simulink model "GeneralFramework"  (R2022a)
settings: Solver=ode23tb  StartTime=0.0  StopTime=t_sim  RelTol=1e-3
values from neighbouring files (symbols this model uses):
  AccPwrbp = [0 3.0779560993538198]    [Init_Parameters.m]
  AccSpdbp = [256.49641719585139 641.24104298962845]    [Init_Parameters.m]
  EngTrqSat = 60    [Init_Parameters.m]
  f_mu = ones(4,1)    [Init_Parameters.m]
  InitialLatPosition = 0    [Init_Parameters.m]
  numWheels = 4    [Init_Parameters.m]    (also in VehicleParameters.m)
  omega_hw = 13.51    [Init_Parameters.m]
  steerDir = -1    [Init_Parameters.m]
  t_start = 1    [Init_Parameters.m]
  t_stop = 100    [Init_Parameters.m]
  theta_max = 270    [Init_Parameters.m]
  TrackWidth = VEH.TrackWidth    [Init_Parameters.m]
  Trans = data.Trans    [Init_Parameters.m]    (also in ModelWorkspace.mat = )
  VEH = data.VEH    [Init_Parameters.m]    (also in ModelWorkspace.mat = ; VehicleParameters.m)
  wheelB = VEH.FrontAxlePositionfromCG+VEH.RearAxlePositionfromCG    [Init_Parameters.m]    (also in VehicleParameters.m)
  xdot_r = 2    [Init_Parameters.m]
libraries: autolibutils x10, simulink x8, sharedtransform x5, autolibsharedcoupling x3, vehdynlibsuspension x2, shared6dof x2, autolibtranscontrolscommon x1, vehdynlibdriver x1, autolibsharedtransfixedgear x1, vehdynlibsteering x1, autolibshareddiff x1, autolibsharedmappedengines x1
(part 1 of 5)
settings Model: Creator=monic  LastModifiedBy=monic
settings DebuggingCC: UnconnectedInputMsg=warning  UnconnectedOutputMsg=warning  UnconnectedLineMsg=warning
settings RTWCC: DLArmComputeVersion=19.05

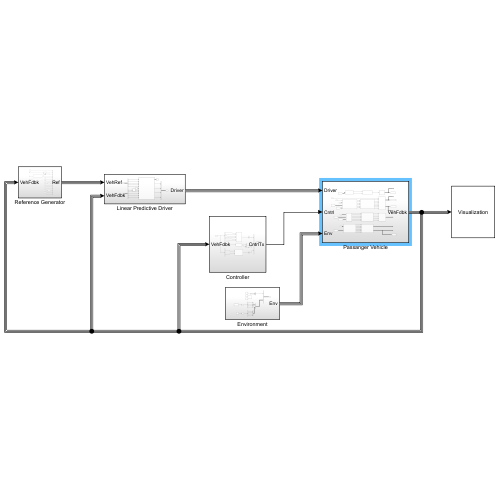
[thumbnail: Simulink's stored preview of the top-level diagram]
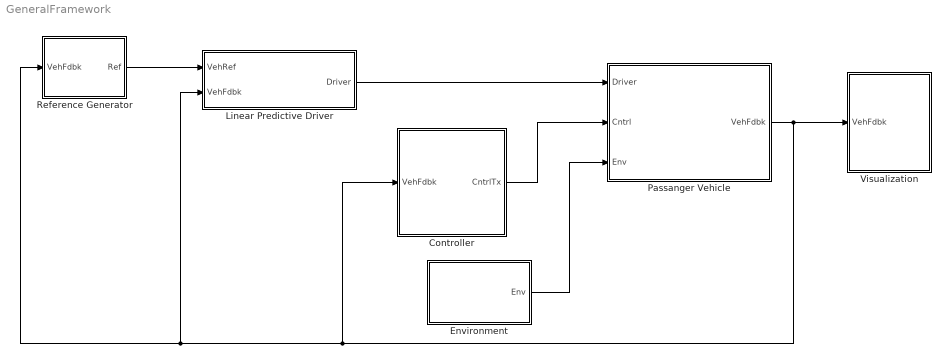
== system GeneralFramework ==
  Controller : Subsystem
  Environment : Subsystem
  Linear Predictive Driver : Subsystem
  Passanger Vehicle : Subsystem
  Reference Generator : Subsystem
  Visualization : Subsystem
      mask Display: disp('Visualization')
  wires:
  Environment/1(Env) -> Passanger Vehicle/3(Env)
  Linear Predictive Driver/1(Driver) -> Passanger Vehicle/1(Driver)
  Passanger Vehicle/1(VehFdbk) -> Visualization/1(VehFdbk), Controller/1(VehFdbk), Linear Predictive Driver/2(VehFdbk), Reference Generator/1(VehFdbk)
  Reference Generator/1(Ref) -> Linear Predictive Driver/1(VehRef)
  Controller/1(CntrlTx) -> Passanger Vehicle/2(Cntrl)

== system GeneralFramework/Controller ==
  VehFdbk : Inport
  Active Differential Control : Subsystem  VariantControl=0
  Brake Pressure Control : Subsystem  VariantControl=0
  Bus Creator1 : BusCreator  Inputs=1
  Bus Creator2 : BusCreator  Inputs=2
  Bus Creator3 : BusCreator  Inputs=3
  Bus Creator4 : BusCreator  Inputs=1
  Bus Selector : BusSelector  OutputSignals=Driver.DecelFdbk
  Bus Selector1 : BusSelector  OutputSignals=Driver.AccFdbk,Driver.DecelFdbk,Driver.GearFdbk,Driveline.EngSpd,Wheels.TireFrame.Omega
  Bus Selector3 : BusSelector  OutputSignals=Driver.AccFdbk,Driver.SteerFdbk
  Trasmission Control : Subsystem
  CntrlTx : Outport  VectorParamsAs1DForOutWhenUnconnected=off
  wires:
  VehFdbk/1 -> Bus Selector3/1, Bus Selector/1, Bus Selector1/1
  Bus Selector1/3 -> Trasmission Control/3(GearReq)  "<GearFdbk>"
  Bus Selector1/4 -> Trasmission Control/4(EngSpd)  "<EngSpd>"
  Bus Selector1/2 -> Trasmission Control/2(BrkCmd)  "<DecelFdbk>"
  Bus Selector1/5 -> Trasmission Control/5(Omega)  "<Omega>"
  Bus Selector/1 -> ?  "<DecelFdbk>"
  Bus Selector1/1 -> Trasmission Control/1(Accel)  "<AccFdbk>"
  [ABSFlag] -> Trasmission Control/6(ABSFlag)
  Bus Selector3/2 -> Active Differential Control/2(Steer)  "<SteerFdbk>"
  Bus Selector3/1 -> Active Differential Control/1(axayaz)  "<AccFdbk>"
  Brake Pressure Control/2(ABSFlag) -> [ABSFlag], Bus Creator2/2  "ABSFlag"
  Brake Pressure Control/1(BrkPrsCmd) -> Bus Creator2/1  "BrkPrsCmd"
  Bus Creator3/1 -> CntrlTx/1  "CntrlTx"
  Trasmission Control/1(Gear) -> Bus Creator1/1  "GearCmd"
  Active Differential Control/1(DiffPrsCmd) -> Bus Creator4/1  "DiffPrsCmd"
  Bus Creator4/1 -> Bus Creator3/3  "Diff"
  Bus Creator1/1 -> Bus Creator3/1  "Transmission"
  Bus Creator2/1 -> Bus Creator3/2  "BrkPrsCmd"

== system GeneralFramework/Environment ==
  Bus Creator : BusCreator  Inputs=4
  Bus Creator1 : BusCreator  Inputs=2
  Bus Creator2 : BusCreator  Inputs=4
  Bus Creator3 : BusCreator  Inputs=2
  Constant1 : Constant  Value=zeros(4,1)
  Constant2 : Constant  Value=f_mu
  Constant3 : Constant  Value=0
  Constant4 : Constant  Value=0
  Constant5 : Constant  Value=0
  Demux : Demux
  Demux1 : Demux
  Signal Specification : SignalSpecification  Unit=m
  Signal Specification1 : SignalSpecification  Unit=1
  Vector Concatenate : Concatenate  NumInputs=3
  Env : Outport  VectorParamsAs1DForOutWhenUnconnected=off
  wires:
  Constant3/1 -> Vector Concatenate/1  "X"
  Constant5/1 -> Vector Concatenate/3  "Z"
  Bus Creator1/1 -> Env/1
  Vector Concatenate/1 -> Bus Creator1/1  "Wind"
  Constant4/1 -> Vector Concatenate/2  "Y"
  Bus Creator3/1 -> Bus Creator1/2  "Ground"
  Demux1/3 -> Bus Creator2/3  "mu_RL"
  Demux1/1 -> Bus Creator2/1  "mu_FL"
  Bus Creator2/1 -> Bus Creator3/2  "mu"
  Demux1/4 -> Bus Creator2/4  "mu_RR"
  Bus Creator/1 -> Bus Creator3/1  "z"
  Demux1/2 -> Bus Creator2/2  "mu_FR"
  Demux/2 -> Bus Creator/2  "G_FR_z"
  Signal Specification1/1 -> Demux1/1
  Demux/3 -> Bus Creator/3  "G_RL_z"
  Demux/4 -> Bus Creator/4  "G_RR_z"
  Demux/1 -> Bus Creator/1  "G_FL_z"
  Signal Specification/1 -> Demux/1
  Constant1/1 -> Signal Specification/1
  Constant2/1 -> Signal Specification1/1

== system GeneralFramework/Linear Predictive Driver ==
  VehRef : Inport
  VehFdbk : Inport  Port=2
  Bus Creator1 : BusCreator  Inputs=4
  Bus Selector : BusSelector  OutputSignals=Body.BdyFrm.Cg.Vel.xdot,Body.InertFrm.Cg.Disp.Y,Body.BdyFrm.Cg.Vel.ydot,Body.InertFrm.Cg.Ang.psi,Body.BdyFrm.Cg.AngVel.r
  Bus Selector1 : BusSelector  OutputSignals=LngRef,LtrlRef,EnblSteerCmd,SteerOvrCmd,AccelZero
  Dead Zone : DeadZone  LowerValue=-.5  UpperValue=.5  ZeroCross=off
  Ground : Ground
  Linear Predictive Driver : vehdynlibdriver/Predictive Driver  extAccelOvr=off  extDecelOvr=off  extAccelHld=off  extDecelHld=off  extAccelZero=on  extDecelZero=off  extSteerOvr=on  extSteerHld=off  extSteerZero=off  cntrlType=Predictive  cntrlTypeLat=Predictive  shftType=Reverse, Neutral, Drive  coordMode=SAE J670 (Z-down)  refType=Reference pose  velUnits=m/s  angUnits=rad  gearOut=on  steerOut=on  Kp=3  Ki=1  Kff=1  Kg=0  VehVelVec=[0 100]  KffVec=[.1 .1]  KpVec=[10 10]  KiVec=[5 5]  KgVec=[0 0]  vnom=5  Kaw=1  tauerr=.075  tau=0.3  L=0.75  Kpt=15000  aR=200  bR=2.5  cR=.5  g=9.81  vecPose=off  dynamMode=off  PositionGainF=2.5  PositionGainR=2.5  YawRateGain=.2  DelayGain=.2  enableDrift=off  BetaRef=20*pi/180  KpBeta=1  KpDrift=2  KdDrift=1  KpPsi=6  KOmega=30  tOmega=1  a=VEH.FrontAxlePositionfromCG  b=VEH.RearAxlePositionfromCG  m=VEH.Mass  Cy_f=50000  Cy_r=70000  I=VEH.YawMomentInertia  Ksteer=18  theta=40*pi/180  Idl=3  Re=.3  lambda_mu=1  GearInit=0  tShift=.1  pdlVec=[0.1 0.4 0.5 0.9]  upShftTbl=[-1 12.9375 26.4375 39.9375 51.18749999999999 62.4375 72.84375 83.25;-1 16.3125 29.8125 43.3125 54.5624 65.8125 76.78125 87.75;-1 19.6875 33.1875 46.68749999999999 57.9375 69.1875 80.71875 92.25;-1 33 52.5 77.25 100.5 138.75 161.875 185]  dwnShftTbl=[-1 12.9375 26.4375 39.9375 51.18749999999999 62.4375 72.84375 83.25;-1 16.3125 29.8125 43.3125 54.5624 65.8125 76.78125 87.75;-1 19.6875 33.1875 46.68749999999999 57.9375 69.1875 80.71875 92.25;-1 33 52.5 77.25 100.5 138.75 161.875 185]  tClutch=.5  tRev=.5  tPark=120  UpGearVec="[0  1  2  3  4  5  6  7]"  DownGearVec="[1  2  3  4  5  6  7  8]"  aMode=2
      settings: SourceProductBaseCode=VE
  Terminator : Terminator
  Driver : Outport
  wires:
  Linear Predictive Driver/4 -> Bus Creator1/3  "DecelCmd"
  Bus Selector/3 -> Linear Predictive Driver/9  "<ydot>"
  Ground/1 -> Linear Predictive Driver/6
  Bus Selector/5 -> Linear Predictive Driver/11  "<r>"
  VehFdbk/1 -> Bus Selector/1
  Bus Selector1/4 -> Linear Predictive Driver/4  "<SteerOvrCmd>"
  Bus Selector/1 -> Dead Zone/1  "<xdot>"
  Bus Selector1/1 -> Linear Predictive Driver/1  "<LngRef>"
  Bus Selector1/2 -> Linear Predictive Driver/2  "<LtrlRef>"
  Linear Predictive Driver/3 -> Bus Creator1/2  "AccelCmd"
  Bus Selector1/3 -> Linear Predictive Driver/3  "<EnblSteerCmd>"
  Linear Predictive Driver/5 -> Bus Creator1/4  "GearCmd"
  Bus Creator1/1 -> Driver/1
  Bus Selector/2 -> Linear Predictive Driver/8  "<Y>"
  Linear Predictive Driver/2 -> Bus Creator1/1  "SteerCmd"
  Bus Selector/4 -> Linear Predictive Driver/10  "<psi>"
  Bus Selector1/5 -> Linear Predictive Driver/5  "<AccelZero>"
  Linear Predictive Driver/1 -> Terminator/1
  Dead Zone/1 -> Linear Predictive Driver/7
  VehRef/1 -> Bus Selector1/1

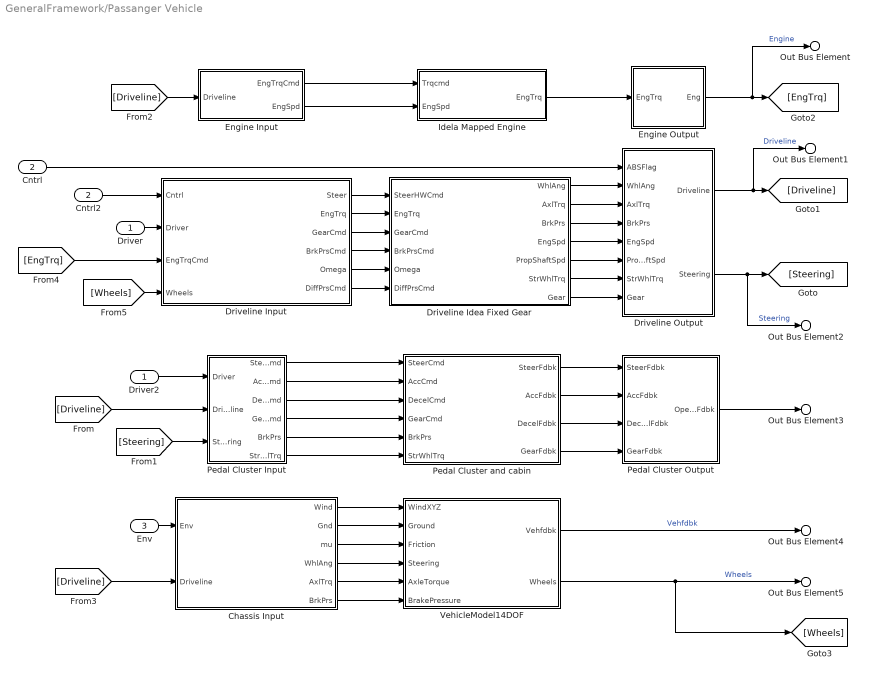
== system GeneralFramework/Passanger Vehicle ==
  Driver : Inport
  Cntrl : Inport  Port=2
  Env : Inport  Port=3
  Chassis Input : Subsystem
  Cntrl2 : InportShadow  Port=2
  Driveline Idea Fixed Gear : Subsystem
  Driveline Input : Subsystem
  Driveline Output : Subsystem
  Driver2 : InportShadow
  Engine Input : Subsystem
  Engine Output : Subsystem
  Idela Mapped Engine : Subsystem
  Pedal Cluster Input : Subsystem
  Pedal Cluster Output : Subsystem
  Pedal Cluster and cabin : Subsystem
  VehicleModel14DOF : Subsystem
  Out Bus Element4 : Outport  PortName=VehFdbk  Element=Body
  Out Bus Element5 : Outport  PortName=VehFdbk  Element=Wheels
  Out Bus Element3 : Outport  PortName=VehFdbk  Element=Driver
  Out Bus Element2 : Outport  PortName=VehFdbk  Element=Steering
  Out Bus Element1 : Outport  PortName=VehFdbk  Element=Driveline
  Out Bus Element : Outport  PortName=VehFdbk  Element=Engine
  wires:
  Driveline Idea Fixed Gear/7(Gear) -> Driveline Output/8(Gear)
  [Driveline] -> Chassis Input/2(Driveline)
  Engine Input/1(EngTrqCmd) -> Idela Mapped Engine/1(Trqcmd)
  Pedal Cluster and cabin/2(AccFdbk) -> Pedal Cluster Output/2(AccFdbk)
  Driveline Input/4(BrkPrsCmd) -> Driveline Idea Fixed Gear/4(BrkPrsCmd)
  Pedal Cluster Input/3(DecelCmd) -> Pedal Cluster and cabin/3(DecelCmd)
  VehicleModel14DOF/2(Wheels) -> Out Bus Element5/1, [Wheels]  "Wheels"
  Pedal Cluster Input/2(AccelCmd) -> Pedal Cluster and cabin/2(AccCmd)
  Driver/1 -> Driveline Input/2(Driver)
  Pedal Cluster and cabin/3(DecelFdbk) -> Pedal Cluster Output/3(DecelFdbk)
  Engine Input/2(EngSpd) -> Idela Mapped Engine/2(EngSpd)
  [Driveline] -> Pedal Cluster Input/2(Driveline)
  Driveline Idea Fixed Gear/1(WhlAng) -> Driveline Output/2(WhlAng)
  Pedal Cluster and cabin/4(GearFdbk) -> Pedal Cluster Output/4(GearFdbk)
  Driveline Input/3(GearCmd) -> Driveline Idea Fixed Gear/3(GearCmd)
  [Steering] -> Pedal Cluster Input/3(Steering)
  Cntrl/1 -> Driveline Output/1(ABSFlag)
  [EngTrq] -> Driveline Input/3(EngTrqCmd)
  Driveline Input/6(DiffPrsCmd) -> Driveline Idea Fixed Gear/6(DiffPrsCmd)
  Driver2/1 -> Pedal Cluster Input/1(Driver)
  Idela Mapped Engine/1(EngTrq) -> Engine Output/1("EngTrq ")
  Pedal Cluster Input/1(SteerCmd) -> Pedal Cluster and cabin/1(SteerCmd)
  Pedal Cluster Input/5(BrkPrs) -> Pedal Cluster and cabin/5(BrkPrs)
  [Wheels] -> Driveline Input/4(Wheels)
  Driveline Input/1(Steer) -> Driveline Idea Fixed Gear/1(SteerHWCmd)
  Driveline Input/2(EngTrq) -> Driveline Idea Fixed Gear/2(EngTrq)
  Pedal Cluster and cabin/1(SteerFdbk) -> Pedal Cluster Output/1(SteerFdbk)
  Driveline Input/5(Omega) -> Driveline Idea Fixed Gear/5(Omega)
  Env/1 -> Chassis Input/1(Env)
  Driveline Idea Fixed Gear/3(BrkPrs) -> Driveline Output/4(BrkPrs)
  Driveline Idea Fixed Gear/4(EngSpd) -> Driveline Output/5(EngSpd)
  Driveline Output/2(Steering) -> Out Bus Element2/1, [Steering]  "Steering"
  Engine Output/1(Eng) -> Out Bus Element/1, [EngTrq]  "Engine"
  Driveline Idea Fixed Gear/6(StrWhlTrq) -> Driveline Output/7(StrWhlTrq)
  Driveline Idea Fixed Gear/5(PropShaftSpd) -> Driveline Output/6(PropShftSpd)
  [Driveline] -> Engine Input/1(Driveline)
  Pedal Cluster Input/4(GearCmd) -> Pedal Cluster and cabin/4(GearCmd)
  Driveline Idea Fixed Gear/2(AxlTrq) -> Driveline Output/3(AxlTrq)
  VehicleModel14DOF/1(Vehfdbk) -> Out Bus Element4/1  "Vehfdbk"
  Pedal Cluster Input/6(StrWhlTrq) -> Pedal Cluster and cabin/6(StrWhlTrq)
  Cntrl2/1 -> Driveline Input/1(Cntrl)
  Pedal Cluster Output/1(OperatorFdbk) -> Out Bus Element3/1
  Driveline Output/1(Driveline) -> Out Bus Element1/1, [Driveline]  "Driveline"
  Chassis Input/1(Wind) -> VehicleModel14DOF/1(WindXYZ)
  Chassis Input/2(Gnd) -> VehicleModel14DOF/2(Ground)
  Chassis Input/3(mu) -> VehicleModel14DOF/3(Friction)
  Chassis Input/4(WhlAng) -> VehicleModel14DOF/4(Steering)
  Chassis Input/5(AxlTrq) -> VehicleModel14DOF/5(AxleTorque)
  Chassis Input/6(BrkPrs) -> VehicleModel14DOF/6(BrakePressure)

== system GeneralFramework/Reference Generator ==
  Bus Element In1 : Inport  PortName=VehFdbk  Element=Body.BdyFrm.Cg.Vel.xdot
  Bus Element In2 : Inport  PortName=VehFdbk  Element=Body.InertFrm.Cg.Disp.Y
  Bus Creator2 : BusCreator  Inputs=14
  Compare To Zero : simulink/Logic and Bit Operations/Compare To Zero  relop=~=  OutDataTypeStr=boolean  ZeroCross=off
  Constant{4..7,10..12} (7 alike) : Constant  Value=false
  Constant2 : Constant  Value=false  OutDataTypeStr=boolean
  Constant3 : Constant  Value=0
  Constant8 : Constant  Value=0
  Ground : Ground
  LatchSwitchCont : autolibutils/LatchSwitchCont  aMode=2
      settings: SourceProductBaseCode=PW,DR,MT,VE
  Longitudinal Velocity Reference : vehdynlibscenariocommon/Slowly Increasing Steer/Longitudinal Velocity Reference  SystemSampleTime=-1  VariantActivationTime=update diagram  Latency=0  AutoFrameSizeCalculation=off
      settings: SourceProductBaseCode=VE
  Signal Specification : SignalSpecification  Unit=m
  Signal Specification2 : SignalSpecification  Unit=one
  Signal Specification3 : SignalSpecification  Unit=one
  Steer Command Generator : Subsystem
  Ref : Outport  VectorParamsAs1DForOutWhenUnconnected=off
  wires:
  Steer Command Generator/1(SteerOvrCmd) -> Compare To Zero/1, Bus Creator2/4  "SteerOvrCmd"
  Signal Specification3/1 -> Bus Creator2/12  "DecelOvrCmd"
  Constant10/1 -> Bus Creator2/11  "EnblDecelCmd"
  Constant4/1 -> Bus Creator2/7  "EnblAccelOvr"
  LatchSwitchCont/1 -> Bus Creator2/3  "EnblSteerCmd"
  Constant8/1 -> Signal Specification2/1
  Signal Specification2/1 -> Bus Creator2/8  "AccelOvrCmd"
  Longitudinal Velocity Reference/1 -> Bus Creator2/1  "LngRef"
  Constant3/1 -> Signal Specification3/1
  Bus Creator2/1 -> Ref/1
  Constant2/1 -> Bus Creator2/10  "AccelZero"
  Constant5/1 -> Bus Creator2/5  "SteerHld"
  Compare To Zero/1 -> LatchSwitchCont/1
  Constant7/1 -> Bus Creator2/9  "AccelHld"
  Signal Specification/1 -> Bus Creator2/2  "LtrlRef"
  Constant6/1 -> Bus Creator2/6  "SteerZero"
  Constant11/1 -> Bus Creator2/13  "DecelHld"
  Constant12/1 -> Bus Creator2/14  "DecelZero"
  Ground/1 -> LatchSwitchCont/2
  Bus Element In1/1 -> Steer Command Generator/1(<xdot>)
  Bus Element In2/1 -> Signal Specification/1

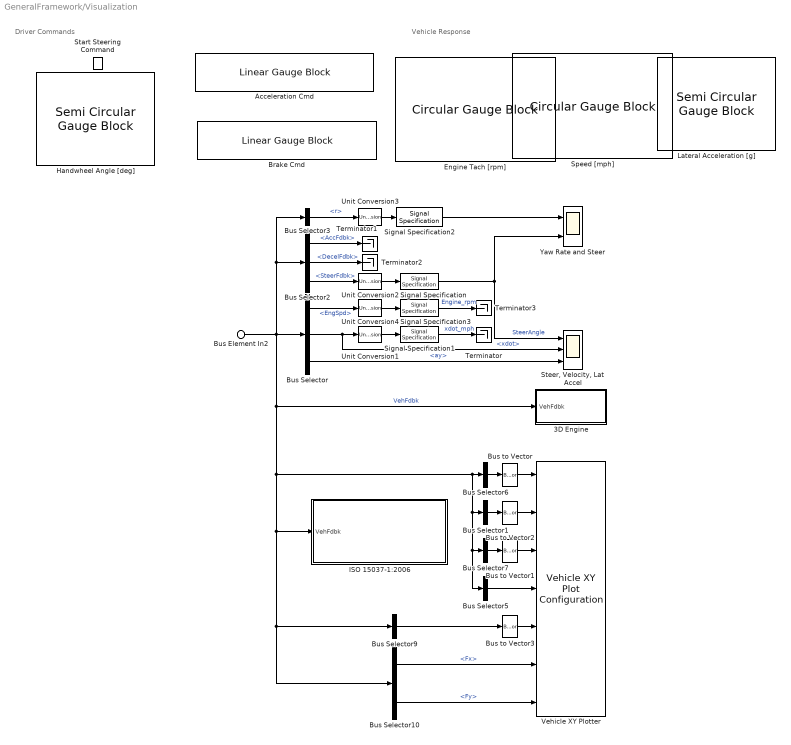
== system GeneralFramework/Visualization ==
  note: Driver Commands
  note: Vehicle Response
  Bus Element In2 : Inport  PortName=VehFdbk
  3D Engine : Subsystem  Variant=on  mask(3D Engine){engine3D=Disabled, use3DOp=off, SceneDesc=Open surface, dt3D=.03, defaultPos=Recommended for scene, X_o=0, Y_o=0, Z_o=0, phi_o=0, theta_o=0, psi_o=0}
      mask prompts: engine3D "vdynblks:vehdynRefApp3DEng:blkPrm_engine3D"; use3DOp "Use default operating point"; SceneDesc "vdynblks:vehdynRefApp3DEng:blkPrm_SceneDesc"; dt3D "vdynblks:vehdynRefApp3DEng:blkPrm_dt3D"; X_o "vdynblks:vehdynRefApp3DEng:blkPrm_X_o"; Y_o "vdynblks:vehdynRefApp3DEng:blkPrm_Y_o"; Z_o "vdynblks:vehdynRefApp3DEng:blkPrm_Z_o"; phi_o "vdynblks:vehdynRefApp3DEng:blkPrm_phi_o"; theta_o "vdynblks:vehdynRefApp3DEng:blkPrm_theta_o"; psi_o "vdynblks:vehdynRefApp3DEng:blkPrm_psi_o"
      mask help: This subsystem contains the interface blocks which permit the display of the vehicle in the 3D virtual environment. Enable it to view the simulation progress, disable it to inhibit the display.
      mask init:
      | GrndFdbkPath = find_system(bdroot(gcb),'BlockType','SubSystem','Name','Ground Feedback');
      | ManBlkName = 'Slowly Increasing Steer';
      | ManBlkPath = find_system(bdroot(gcb),'BlockType','SubSystem','Name',ManBlkName);
      | OpVarName = 'dlcSS35mph';
      | switch get_param(gcb,'engine3D')    
      |     case 'Disabled'
      |         try
      |             set_param(GrndFdbkPath{:},'OverrideUsingVariant','0');
      |         catch
      |             disp('Warning: No ground feedback sensor not set')
      |         end
      |         try
      |             if strcmp(get_param(gcb,'use3DOp'),'on') && strcmp(get_param(ManBlkPath{:},'ssMode'),'Resume from a workspace variable')
      |                 set_param(ManBlkPath{:},'ssVar',OpVarName);
      |             end
      |         catch
      |              disp('Warning: Maneuver source block not found. Steady state operating point not set')
      |         end
      |     case 'Enabled'
      |         try
      |             set_param(GrndFdbkPath{:},'OverrideUsingVariant','1');            
      |         catch
      |             disp('Warning: Ground feedback from game engine was not found. Using constant values from model instead.')
      |         end
      |         try
      |             if strcmp(get_param(gcb,'use3DOp'),'on') && strcmp(get_param(ManBlkPath{:},'ssMode'),'Resume from a workspace variable')
      |                 set_param(ManBlkPath{:},'ssVar',[OpVarName '3D']);
      |             end
      |         catch
      |              disp('Warning: Maneuver source block not found. Steady state operating point not set')
      |         end
      |     otherwise
      | end
      settings: AttributesFormatString=|
      | %<SceneDesc>
      | %<engine3D>
      mask Help: eval('vdynblkshelp(''vdynblks3dengine'')');
      mask TypeOptions engine3D: Enabled | Disabled
      mask Callback engine3D:
      | switch get_param(gcb,'engine3D')
      |     case 'Disabled'
      |         try
      |             % add specifics here if needed
      |         catch
      |             disp('Warning: Maneuver source block not found in model')
      |         end
      |     case 'Enabled'
      |         try
      |             % add specifics here if needed
      |         catch
      |             disp('Warning: Maneuver source block not found in model')
      |         end
      |     otherwise
      | end
      mask TypeOptions SceneDesc: 3D Engine/Simulation 3D Scene Configuration/SceneDesc
      mask Callback SceneDesc:
      | defaultStatus = get_param(gcb,'defaultPos');
      | if strcmp(defaultStatus,'Recommended for scene')
      | sceneType = get_param(gcb,'SceneDesc');
      | switch sceneType
      |     case 'Straight road'
      |         set_param(gcb,'X_o', '-118')
      |         set_param(gcb,'Y_o', '3.125')
      |         set_param(gcb,'Z_o', '0')
      |         set_param(gcb,'phi_o', '0')
      |         set_param(gcb,'theta_o', '0')
      |         set_param(gcb,'psi_o', '0')
      |     case 'Curved road'
      |         set_param(gcb,'X_o', '0.2')
      |         set_param(gcb,'Y_o', '-1605.0')
      |         set_param(gcb,'Z_o', '0')
      |         set_param(gcb,'phi_o', '0')
      |         set_param(gcb,'theta_o', '0')
      |         set_param(gcb,'psi_o', '-156*pi/180')
      |     case 'Parking lot'
      |         set_param(gcb,'X_o', '-104.0')
      |         set_param(gcb,'Y_o', '-9.7')
      |         set_param(gcb,'Z_o', '0')
      |         set_param(gcb,'phi_o', '0')
      |         set_param(gcb,'theta_o', '0')
      |         set_param(gcb,'psi_o', '0')
      |     case 'Double lane change'
      |         set_param(gcb,'X_o', '0')
      |         set_param(gcb,'Y_o', '3.125')
      |         set_param(gcb,'Z_o', '0')
      |         set_param(gcb,'phi_o', '0')
      |         set_param(gcb,'theta_o', '0')
      |         set_param(gcb,'psi_o', '0')
      |     case 'Open surface'
      |         set_param(gcb,'X_o', '0')
      |         set_param(gcb,'Y_o', '0')
      |         set_param(gcb,'Z_o', '0')
      |         set_param(gcb,'phi_o', '0')
      |         set_param(gcb,'theta_o', '0')
      |         set_param(gcb,'psi_o', '0')
      |     case 'US highway'
      |         set_param(gcb,'X_o', '3592.00')
      |         set_param(gcb,'Y_o', '2617.00')
      |         set_param(gcb,'Z_o', '-1.0')
      |         set_param(gcb,'phi_o', '0')
      |         set_param(gcb,'theta_o', '0')
      |         set_param(gcb,'psi_o', '0')
      |     case 'US city block'
      |         set_param(gcb,'X_o', '-125.19')
      |         set_param(gcb,'Y_o', '1.65')
      |         set_param(gcb,'Z_o', '-0.04')
      |         set_param(gcb,'phi_o', '0')
      |         set_param(gcb,'theta_o', '0')
      |         set_param(gcb,'psi_o', '0')
      |     case 'Large parking lot'
      |         set_param(gcb,'X_o', '45.0')
      |         set_param(gcb,'Y_o', '54.7')
      |         set_param(gcb,'Z_o', '0.0')
      |         set_param(gcb,'phi_o', '0')
      |         set_param(gcb,'theta_o', '0')
      |         set_param(gcb,'psi_o', '-pi/2')
      |     case 'Virtual Mcity'
      |         set_param(gcb,'X_o', '-26.0')
      |         set_param(gcb,'Y_o', '76.0')
      |         set_param(gcb,'Z_o', '0.0')
      |         set_param(gcb,'phi_o', '0')
      |         set_param(gcb,'theta_o', '0')
      |         set_param(gcb,'psi_o', '-40*pi/180')
      |     otherwise
      |         set_param(gcb,'X_o', '0')
      |         set_param(gcb,'Y_o', '0')
      |         set_param(gcb,'Z_o', '0')
      |         set_param(gcb,'phi_o', '0')
      |         set_param(gcb,'theta_o', '0')
      |         set_param(gcb,'psi_o', '0')
      | end
      | end
      mask TypeOptions defaultPos: Recommended for scene | User-specified
      mask DialogControl engineConfig Prompt: vdynblks:vehdynRefApp3DEng:blkDlg_engineConfig
      mask DialogControl engine3D Prompt: 3D Engine
      mask DialogControl SceneDesc Prompt: Scene:
      mask DialogControl dt3D Prompt: 3D Engine frame rate, dt3D [s]:
      mask DialogControl posSetup Prompt: vdynblks:vehdynRefApp3DEng:blkDlg_posSetup
      mask DialogControl posSetupDesc Prompt: vdynblks:vehdynRefApp3DEng:blkDisTxt_posSetupDesc
      mask DialogControl X_o Prompt: Initial longitudinal position, X_o [m]:
      mask DialogControl Y_o Prompt: Initial lateral position, Y_o [m]:
      mask DialogControl Z_o Prompt: Initial vertical position, Z_o [m]:
      mask DialogControl phi_o Prompt: Initial roll angle, phi_o [rad]:
      mask DialogControl theta_o Prompt: Initial pitch angle, theta_o [rad]:
      mask DialogControl psi_o Prompt: Initial yaw angle, psi_o [rad]:
      mask DialogControl setModelPos Prompt: vdynblks:vehdynRefApp3DEng:blkDlg_setModelPos
      mask DialogControl setModelPos Callback:
      | if strcmp(get_param(bdroot(gcb),'SimulationStatus'),'stopped')
      |     sceneType = get_param(gcb,'SceneDesc');
      |     rootModel = bdroot(gcb);
      |     ws = get_param(rootModel, 'modelworkspace');
      |     VEH = getVariable(ws,'VEH');
      |     ParamList={'X_o',[1,1],{};'Y_o',[1,1],{};'Z_o',[1,1],{};'phi_o',[1,1],{'gte',-pi/2;'lte',pi/2};'theta_o',[1,1],{'gte',-pi/2;'lte',pi/2};'psi_o',[1,1],{'gte',-2*pi;'lte',2*pi}};
      |     paramStruct = autoblkscheckparams(gcb, '3D Engine',ParamList);
      |     VEH.InitialLongPosition = paramStruct.X_o;
      |     VEH.InitialLatPosition = paramStruct.Y_o;
      |     VEH.InitialVertPosition = paramStruct.Z_o;
      |     VEH.InitialRollAngle = paramStruct.phi_o;
      |     VEH.InitialPitchAngle = paramStruct.theta_o;
      |     VEH.InitialYawAngle = paramStruct.psi_o;
      |     assignin(ws,'VEH',VEH);
      |     modelList = {'PassVeh14DOF','PassVeh7DOF'};
      |     for idx =1:length(modelList)
      | %         try
      |             load_system(modelList{idx});
      |             ws = get_param(modelList{idx}, 'modelworkspace');
      |             assignin(ws,'VEH',VEH);
      |             save_system(modelList{idx});
      |             close_system(modelList{idx});
      | %         catch
      | %             disp(['Cannot find ' modelList{idx}])
      | %         end
      |     end
      | end
      mask Display: disp('3D Engine')
  Acceleration Cmd : LinearGaugeBlock  LabelPosition=Hide  ScaleMax=1  TickInterval=0.20000000000000001
  Brake Cmd : LinearGaugeBlock  LabelPosition=Hide  ScaleMax=1  TickInterval=0.20000000000000001
  Bus Selector : BusSelector  OutputSignals=Driveline.EngSpd,Body.BdyFrm.Cg.Vel.xdot,Body.BdyFrm.Cg.Acc.ay
  Bus Selector1 : BusSelector  OutputSignals=Body.InertFrm.Cg.Ang.phi,Body.InertFrm.Cg.Ang.theta,Body.InertFrm.Cg.Ang.psi  OutputAsBus=on
  Bus Selector10 : BusSelector  OutputSignals=Wheels.TireFrame.Fx,Wheels.TireFrame.Fy
  Bus Selector2 : BusSelector  OutputSignals=Driver.AccFdbk,Driver.DecelFdbk,Driver.SteerFdbk
  Bus Selector3 : BusSelector  OutputSignals=Body.BdyFrm.Cg.AngVel.r
  Bus Selector5 : BusSelector  OutputSignals=Driveline.WhlAng  OutputAsBus=on
  Bus Selector6 : BusSelector  OutputSignals=Body.InertFrm.Geom.Disp.X,Body.InertFrm.Geom.Disp.Y,Body.InertFrm.Geom.Disp.Z  OutputAsBus=on
  Bus Selector7 : BusSelector  OutputSignals=Body.InertFrm.Geom.Vel.Xdot,Body.InertFrm.Geom.Vel.Ydot,Body.InertFrm.Geom.Vel.Zdot  OutputAsBus=on
  Bus Selector9 : BusSelector  OutputSignals=Driveline.EngSpd,Driveline.Gear  OutputAsBus=on
  Bus to Vector{,1..3} (4 alike) : BusToVector
  Engine Tach [rpm] : CircularGaugeBlock  LabelPosition=Hide  ScaleMax=8000  TickInterval=1000
  Handwheel Angle [deg] : SemiCircularGaugeBlock  LabelPosition=Hide  ScaleMin=-300  ScaleMax=300  TickInterval=60
  ISO 15037-1:2006 : Subsystem  StopFcn=|  Variant=on  VariantControlMode=label  LabelModeActiveChoice=0  mask(ISO 15037-1:2006){Measurement=Disabled}
      | switch get_param(gcb,'Measurement')
      |     case 'Enabled'
      |        p=slproject.getCurrentProject;
      |        projectRoot=p.RootFolder;
      |        SySFolder=fullfile(projectRoot, 'System');
      |        Simulink.sdi.loadView([SySFolder filesep 'ISO15037_1_2006E.mldatx']);
      |        Simulink.sdi.view;
      | end
      mask prompts: Measurement "ISO Measurements"
      mask help: Enables display of ISO 15037-1:2006 standard measurement signals in the Simulation Data Inspector.
      mask init:
      | switch get_param(gcb,'Measurement')
      |     case 'Disabled'
      |         set_param(gcb,'OverrideUsingVariant','0')
      |     case 'Enabled'
      |        set_param(gcb,'OverrideUsingVariant','1')
      |     otherwise
      |        set_param(gcb,'OverrideUsingVariant','0')
      | end
      settings: AttributesFormatString=%<Measurement>
      mask Help: eval('vdynblkshelp(''iso15037'')');
      mask TypeOptions Measurement: Enabled | Disabled
      mask Callback Measurement:
      | switch get_param(gcb,'Measurement')
      |     case 'Disabled'
      |         set_param(gcb,'OverrideUsingVariant','0')
      |     case 'Enabled'
      |        set_param(gcb,'OverrideUsingVariant','1')
      |     otherwise
      |        set_param(gcb,'OverrideUsingVariant','0')
      | end
      mask Display: disp('ISO 15037-1:2006')
  Lateral Acceleration [g] : SemiCircularGaugeBlock  LabelPosition=Hide  ScaleMin=-1  ScaleMax=1  TickInterval=0.5
  Signal Specification : SignalSpecification  Unit=deg
  Signal Specification1 : SignalSpecification  Unit=mph
  Signal Specification2 : SignalSpecification  Unit=deg/s
  Signal Specification3 : SignalSpecification  Unit=rpm
  Speed [mph] : CircularGaugeBlock  LabelPosition=Hide  TickInterval=10
  Start Steering Command : LampBlock  LabelPosition=Hide
  "Steer, Velocity, Lat Accel" : Scope  NumInputPorts=3
  Terminator{,1..3} (4 alike) : Terminator
  Unit Conversion{1..4} (4 alike) : UnitConversion
  Vehicle XY Plotter : vehdynlibviscommon/Vehicle XY Plot Configuration  extRef=off  extStats=on  extTireF=on  a=VEH.FrontAxlePositionfromCG  b=VEH.RearAxlePositionfromCG  w=VEH.TrackWidth  figBorder=10  bufferSize=1024  velNorm=5  tireFNorm=1000  pltDT=.1
      settings: SourceProductBaseCode=VE
  Yaw Rate and Steer : Scope  NumInputPorts=2
  wires:
  Unit Conversion3/1 -> Signal Specification2/1
  Bus Selector3/1 -> Unit Conversion3/1  "<r>"
  Signal Specification2/1 -> Yaw Rate and Steer/1
  Bus to Vector3/1 -> Vehicle XY Plotter/5
  Bus Selector5/1 -> Vehicle XY Plotter/4
  Bus Selector/3 -> "Steer, Velocity, Lat Accel"/3  "<ay>"
  Signal Specification3/1 -> Terminator3/1  "Engine_rpm"
  Bus Selector9/1 -> Bus to Vector3/1
  Bus Element In2/1 -> 3D Engine/1(VehFdbk), Bus Selector10/1, Bus Selector9/1, ISO 15037-1:2006/1(VehFdbk), Bus Selector5/1, Bus Selector7/1, Bus Selector1/1, Bus Selector6/1, Bus Selector3/1, Bus Selector2/1, Bus Selector/1  "VehFdbk"
  Bus Selector2/2 -> Terminator2/1  "<DecelFdbk>"
  Bus to Vector2/1 -> Vehicle XY Plotter/2
  Bus Selector6/1 -> Bus to Vector/1
  Bus to Vector/1 -> Vehicle XY Plotter/1
  Bus Selector1/1 -> Bus to Vector2/1
  Bus to Vector1/1 -> Vehicle XY Plotter/3
  Bus Selector7/1 -> Bus to Vector1/1
  Unit Conversion4/1 -> Signal Specification3/1
  Bus Selector/1 -> Unit Conversion4/1  "<EngSpd>"
  Bus Selector2/1 -> Terminator1/1  "<AccFdbk>"
  Bus Selector2/3 -> Unit Conversion2/1  "<SteerFdbk>"
  Bus Selector10/2 -> Vehicle XY Plotter/7  "<Fy>"
  Signal Specification1/1 -> Terminator/1  "xdot_mph"
  Unit Conversion1/1 -> Signal Specification1/1
  Signal Specification/1 -> Yaw Rate and Steer/2, "Steer, Velocity, Lat Accel"/1  "SteerAngle"
  Bus Selector10/1 -> Vehicle XY Plotter/6  "<Fx>"
  Unit Conversion2/1 -> Signal Specification/1
  Bus Selector/2 -> "Steer, Velocity, Lat Accel"/2, Unit Conversion1/1  "<xdot>"

== system GeneralFramework/Controller/Active Differential Control ==
  axayaz : Inport
  Steer : Inport  Port=2
  Constant : Constant  Value=0
  Terminator : Terminator
  Terminator1 : Terminator
  Vector Concatenate2 : Concatenate  NumInputs=4
  DiffPrsCmd : Outport  VectorParamsAs1DForOutWhenUnconnected=off
  wires:
  Constant/1 -> Vector Concatenate2/1, Vector Concatenate2/4, Vector Concatenate2/3, Vector Concatenate2/2
  Steer/1 -> Terminator1/1
  Vector Concatenate2/1 -> DiffPrsCmd/1  "DiffPrsCmd"
  axayaz/1 -> Terminator/1

== system GeneralFramework/Controller/Brake Pressure Control ==
  Constant : Constant  Value=false
  Constant1 : Constant  Value=zeros(4,1)
  Selector : Selector  InputPortWidth=1  IndexOptions=Index vector (dialog)  Indices=[1 1 1 1]  OutputSizes=1
  BrkPrsCmd : Outport  VectorParamsAs1DForOutWhenUnconnected=off
  ABSFlag : Outport  Port=2
  wires:
  Constant/1 -> Selector/1
  Selector/1 -> ABSFlag/1
  Constant1/1 -> BrkPrsCmd/1  "BrkPrsCmd"

== system GeneralFramework/Controller/Trasmission Control ==
  Accel : Inport
  BrkCmd : Inport  Port=2
  GearReq : Inport  Port=3
  EngSpd : Inport  Port=4  Unit=rad/s
  Omega : Inport  Port=5  Unit=rad/s
  ABSFlag : Inport  Port=6
  Cont LPF : autolibutils/Cont LPF  wc=4*2*pi  AbsoluteTolerance=auto  aMode=2
      settings: SourceProductBaseCode=PW,DR,MT,VE
  Cont LPF1 : autolibutils/Cont LPF  wc=4*2*pi  AbsoluteTolerance=auto  aMode=2
      settings: SourceProductBaseCode=PW,DR,MT,VE
  Gain : Gain  Gain=.3065/4
  OR : Logic  Operator=OR  Inputs=1  AllPortsSameDT=off  OutDataTypeStr=boolean
  Signal Specification : SignalSpecification  Unit=rpm
  Signal Specification1 : SignalSpecification  Unit=m/s
  Sum of Elements : Sum  Inputs=+
  Transmission Controller PRNDL : autolibtranscontrolscommon/Transmission Controller PRNDL  GearInit=1  LugSpd=1200  MinUpSpd=2000  tClutchUp=0.5  tClutchDn=0.5  tPark=120  VelUnit=km/hr  UpShSpd=[20 35 40 50 60 70 85; 25 45 55 60 65 75 85; 30 40 55 65 80 120 150; 45 55 65 75 90 150 185]  UpLdBpt=[.1 .4 .75 1]  UpShBpt=1:7  DnShSpd=[10 15 25 30 40 55 75; 10 18 25 35 50 65 80; 12 18 21 55 65 75 85; 15 20 25 55 70 80 95]  DnLdBpt=[.1 .4 .75 1]  DnShBpt=2:8  POFS=zeros(4,1)  GOFS=zeros(1,7)  Ngears=8  aMode=2
      settings: SourceProductBaseCode=PW,DR,MT,VE
  Gear : Outport  VectorParamsAs1DForOutWhenUnconnected=off
  wires:
  Transmission Controller PRNDL/1 -> Gear/1
  Omega/1 -> Sum of Elements/1
  OR/1 -> Transmission Controller PRNDL/6
  Sum of Elements/1 -> Gain/1
  EngSpd/1 -> Signal Specification/1
  ABSFlag/1 -> OR/1
  Signal Specification1/1 -> Transmission Controller PRNDL/4
  Cont LPF/1 -> Transmission Controller PRNDL/5
  GearReq/1 -> Transmission Controller PRNDL/1  "PRNDL"
  Gain/1 -> Cont LPF1/1
  Cont LPF1/1 -> Signal Specification1/1
  BrkCmd/1 -> Transmission Controller PRNDL/3
  Accel/1 -> Transmission Controller PRNDL/2
  Signal Specification/1 -> Cont LPF/1  "EngSpd"

== system GeneralFramework/Passanger Vehicle/Chassis Input ==
  Env : Inport
  Driveline : Inport  Port=2
  Bus Selector1 : BusSelector  OutputSignals=Ground.z.G_FL_z,Ground.z.G_FR_z,Ground.z.G_RL_z,Ground.z.G_RR_z
  Bus Selector2 : BusSelector  OutputSignals=Wind
  Bus Selector3 : BusSelector  OutputSignals=Ground.mu.mu_FL,Ground.mu.mu_FR,Ground.mu.mu_RL,Ground.mu.mu_RR
  Bus Selector4 : BusSelector  OutputSignals=WhlAng,AxlTrq,BrkPrs
  Scope : Scope
  Vector Concatenate : Concatenate  NumInputs=4
  Vector Concatenate1 : Concatenate  NumInputs=4
  Wind : Outport  VectorParamsAs1DForOutWhenUnconnected=off
  Gnd : Outport  Port=2  VectorParamsAs1DForOutWhenUnconnected=off
  mu : Outport  Port=3  VectorParamsAs1DForOutWhenUnconnected=off
  WhlAng : Outport  Port=4  VectorParamsAs1DForOutWhenUnconnected=off
  AxlTrq : Outport  Port=5  VectorParamsAs1DForOutWhenUnconnected=off
  BrkPrs : Outport  Port=6  VectorParamsAs1DForOutWhenUnconnected=off
  wires:
  Env/1 -> Bus Selector3/1, Bus Selector1/1, Bus Selector2/1
  Bus Selector2/1 -> Wind/1  "<Wind>"
  Bus Selector3/1 -> Vector Concatenate/1  "<mu_FL>"
  Bus Selector3/2 -> Vector Concatenate/2  "<mu_FR>"
  Bus Selector3/3 -> Vector Concatenate/3  "<mu_RL>"
  Bus Selector3/4 -> Vector Concatenate/4  "<mu_RR>"
  Vector Concatenate/1 -> mu/1
  Bus Selector1/1 -> Vector Concatenate1/1  "<G_FL_z>"
  Bus Selector1/2 -> Vector Concatenate1/2  "<G_FR_z>"
  Bus Selector1/3 -> Vector Concatenate1/3  "<G_RL_z>"
  Bus Selector1/4 -> Vector Concatenate1/4  "<G_RR_z>"
  Vector Concatenate1/1 -> Gnd/1
  Driveline/1 -> Bus Selector4/1
  Bus Selector4/2 -> Scope/1, AxlTrq/1  "<AxlTrq>"
  Bus Selector4/1 -> WhlAng/1  "<WhlAng>"
  Bus Selector4/3 -> BrkPrs/1  "<BrkPrs>"

== system GeneralFramework/Passanger Vehicle/Driveline Idea Fixed Gear ==
  SteerHWCmd : Inport
  EngTrq : Inport  Port=2
  GearCmd : Inport  Port=3
  BrkPrsCmd : Inport  Port=4  PortDimensions=4
  Omega : Inport  Port=5
  DiffPrsCmd : Inport  Port=6
  Brake Hydraulics : Subsystem
  Bus Selector : BusSelector  OutputSignals=Trans.TransGear
  Idea Trasmission : Subsystem
  Kinemartic stee : Subsystem
  Rear wheel Active differential : Subsystem
  WhlAng : Outport  Unit=rad  VectorParamsAs1DForOutWhenUnconnected=off
  AxlTrq : Outport  Port=2  VectorParamsAs1DForOutWhenUnconnected=off
  BrkPrs : Outport  Port=3  PortDimensions=4  VectorParamsAs1DForOutWhenUnconnected=off
  EngSpd : Outport  Port=4  VectorParamsAs1DForOutWhenUnconnected=off
  PropShaftSpd : Outport  Port=5  VectorParamsAs1DForOutWhenUnconnected=off
  StrWhlTrq : Outport  Port=6  Unit=N*m  VectorParamsAs1DForOutWhenUnconnected=off
  Gear : Outport  Port=7
  wires:
  Rear wheel Active differential/1(PromptShaftSpd) -> AxlTrq/1
  Omega/1 -> Rear wheel Active differential/2(Omega)
  Rear wheel Active differential/2(DriveshftSpd) -> PropShaftSpd/1, Idea Trasmission/3(CSpd)
  Idea Trasmission/3(CTrq) -> Rear wheel Active differential/1(DriveshftTrq)
  DiffPrsCmd/1 -> Rear wheel Active differential/3(DiffPrsCmd)
  Brake Hydraulics/1(BrkPrs) -> BrkPrs/1
  Idea Trasmission/2(EngSpd) -> EngSpd/1
  BrkPrsCmd/1 -> Brake Hydraulics/1(BrkPrsCmd)
  GearCmd/1 -> Idea Trasmission/1(Gear)
  SteerHWCmd/1 -> Kinemartic stee/1(AngIn)
  Idea Trasmission/1(Info) -> Bus Selector/1
  Kinemartic stee/2(StrWhlTrq) -> StrWhlTrq/1
  Kinemartic stee/1(WhlAng) -> WhlAng/1
  EngTrq/1 -> Idea Trasmission/2(EngTrq)
  Bus Selector/1 -> Gear/1  "<TransGear>"

== system GeneralFramework/Passanger Vehicle/Driveline Input ==
  Cntrl : Inport
  Driver : Inport  Port=2
  EngTrqCmd : Inport  Port=3
  Wheels : Inport  Port=4
  Bus Selector1 : BusSelector  OutputSignals=SteerCmd
  Bus Selector2 : BusSelector  OutputSignals=TireFrame.Omega
  Bus Selector3 : BusSelector  OutputSignals=Transmission.GearCmd,BrkPrsCmd.BrkPrsCmd,Diff.DiffPrsCmd
  Bus Selector4 : BusSelector  OutputSignals=EngTrq
  Data Type Conversion : DataTypeConversion  SaturateOnIntegerOverflow=off  RndMeth=Floor
  Steer : Outport  VectorParamsAs1DForOutWhenUnconnected=off
  EngTrq : Outport  Port=2  VectorParamsAs1DForOutWhenUnconnected=off
  GearCmd : Outport  Port=3  VectorParamsAs1DForOutWhenUnconnected=off
  BrkPrsCmd : Outport  Port=4  VectorParamsAs1DForOutWhenUnconnected=off
  Omega : Outport  Port=5  VectorParamsAs1DForOutWhenUnconnected=off
  DiffPrsCmd : Outport  Port=6  VectorParamsAs1DForOutWhenUnconnected=off
  wires:
  Bus Selector3/1 -> Data Type Conversion/1  "<GearCmd>"
  Driver/1 -> Bus Selector1/1
  Wheels/1 -> Bus Selector2/1
  Bus Selector2/1 -> Omega/1  "<Omega>"
  EngTrqCmd/1 -> Bus Selector4/1
  Bus Selector1/1 -> Steer/1  "<SteerCmd>"
  Bus Selector4/1 -> EngTrq/1  "<EngTrq>"
  Cntrl/1 -> Bus Selector3/1
  Data Type Conversion/1 -> GearCmd/1
  Bus Selector3/2 -> BrkPrsCmd/1  "<BrkPrsCmd>"
  Bus Selector3/3 -> DiffPrsCmd/1  "<DiffPrsCmd>"

== system GeneralFramework/Passanger Vehicle/Driveline Output ==
  ABSFlag : Inport
  WhlAng : Inport  Port=2
  AxlTrq : Inport  Port=3
  BrkPrs : Inport  Port=4
  EngSpd : Inport  Port=5
  PropShftSpd : Inport  Port=6
  StrWhlTrq : Inport  Port=7
  Gear : Inport  Port=8
  Bus Creator1 : BusCreator  Inputs=7
  Bus Creator2 : BusCreator  Inputs=1
  Driveline : Outport  VectorParamsAs1DForOutWhenUnconnected=off
  Steering : Outport  Port=2  VectorParamsAs1DForOutWhenUnconnected=off
  wires:
  Bus Creator1/1 -> Driveline/1  "Driveline"
  PropShftSpd/1 -> Bus Creator1/5  "PropShftSpd"
  AxlTrq/1 -> Bus Creator1/2  "AxlTrq"
  WhlAng/1 -> Bus Creator1/1  "WhlAng"
  EngSpd/1 -> Bus Creator1/4  "EngSpd"
  BrkPrs/1 -> Bus Creator1/3  "BrkPrs"
  StrWhlTrq/1 -> Bus Creator2/1  "StrWhlTrq"
  Bus Creator2/1 -> Steering/1  "Steering"
  Gear/1 -> Bus Creator1/6  "Gear"
  ABSFlag/1 -> Bus Creator1/7  "ABSFlag"

== system GeneralFramework/Passanger Vehicle/Engine Input ==
  Driveline : Inport
  Bus Selector1 : BusSelector  OutputSignals=EngSpd
  Ramp : simulink/Sources/Ramp  slope=5  start=0  InitialOutput=0
  Saturation : Saturate  UpperLimit=EngTrqSat  LowerLimit=0
  Scope : Scope  Commented=on
  To Workspace : ToWorkspace  VariableName=EngTrqCmd  SampleTime=-1
      settings: Save2DSignal=2-D array (concatenate along first dimension)
  EngTrqCmd : Outport  VectorParamsAs1DForOutWhenUnconnected=off
  EngSpd : Outport  Port=2  VectorParamsAs1DForOutWhenUnconnected=off
  wires:
  Driveline/1 -> Bus Selector1/1
  Bus Selector1/1 -> EngSpd/1  "<EngSpd>"
  Ramp/1 -> Saturation/1
  Saturation/1 -> EngTrqCmd/1, To Workspace/1, Scope/1

== system GeneralFramework/Passanger Vehicle/Engine Output ==
  "EngTrq " : Inport
  Bus Creator : BusCreator  Inputs=1
  Eng : Outport  VectorParamsAs1DForOutWhenUnconnected=off
  wires:
  "EngTrq "/1 -> Bus Creator/1  "EngTrq"
  Bus Creator/1 -> Eng/1
